simulink library "simgens"  (Simulink 6.0)
settings: Solver=ode45  StartTime=0.0  StopTime=10.0  RelTol=1e-3
model workspace (MAT data in the model file):
  libCache.blocksTree = {{'simgens', {'Band-Limited White Noise'; 'Chirp Signal'; 'Clock'; 'Constant'; 'Counter Free-Running'; 'Counter Limited'; 'Digital Clock'; 'From File'; 'From Workspace'; 'Ground'; 'Pulse Generator'; 'Ramp'; 'Random Number'; 'Repeating Sequence'; 'Repeating Sequence Interpolated'; 'Repeating Sequence Stair'; 'Signal Builder'; 'Signal Generator'; 'Sine Wave'; 'Step'; 'Uniform Random Number'}}}
  libCache.blockNames{1} = 'simgens'
  libCache.blockNames{2} = 'simgens/Band-Limited
    | White Noise'
  libCache.blockNames{3} = 'simgens/Chirp Signal'
  libCache.blockNames{4} = 'simgens/Clock'
  libCache.blockNames{5} = 'simgens/Constant'
  libCache.blockNames{6} = 'simgens/Counter
    | Free-Running'
  libCache.blockNames{7} = 'simgens/Counter
    | Limited'
  libCache.blockNames{8} = 'simgens/Digital Clock'
  libCache.blockNames{9} = 'simgens/From File'
  libCache.blockNames{10} = 'simgens/From
    | Workspace'
  libCache.blockNames{11} = 'simgens/Ground'
  libCache.blockNames{12} = 'simgens/Pulse
    | Generator'
  libCache.blockNames{13} = 'simgens/Ramp'
  libCache.blockNames{14} = 'simgens/Random
    | Number'
  libCache.blockNames{15} = 'simgens/Repeating
    | Sequence'
  libCache.blockNames{16} = 'simgens/Repeating
    | Sequence
    | Interpolated'
  libCache.blockNames{17} = 'simgens/Repeating
    | Sequence
    | Stair'
  libCache.blockNames{18} = 'simgens/Signal Builder'
  libCache.blockNames{19} = 'simgens/Signal
    | Generator'
  libCache.blockNames{20} = 'simgens/Sine Wave'
  libCache.blockNames{21} = 'simgens/Step'
  libCache.blockNames{22} = 'simgens/Uniform Random
    | Number'
undefined symbols (not defined in the file or in its folder): sigbuilder_block
libraries: simulink x8
PreSaveFcn:
  | iomanager('UpdateCache',bdroot(gcs))
settings Model: LibraryType=IOLibrary  Creator=weis  LastModifiedBy=andyb  ExtModeAutoUpdateStatusClock=off
settings DataIOCC: SignalLoggingName=logsOut
settings DebuggingCC: CheckExecutionContextPreStartOutputMsg=on  CheckExecutionContextRuntimeOutputMsg=on
settings SFSimCC: SFSimApplyToAllLibs=on  SFSimBuildMode=Incremental

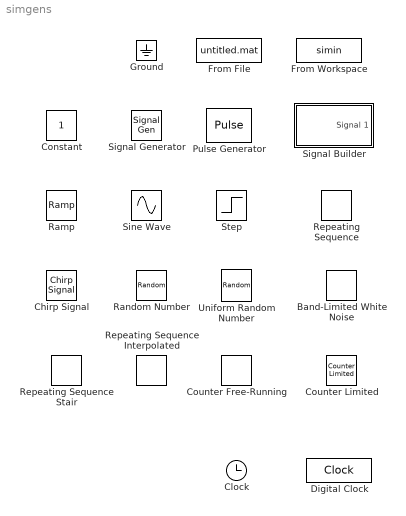
== system simgens ==
  Band-Limited White Noise : simulink/Sources/Band-Limited White Noise  IOType=siggen  Cov=[0.1]  Ts=0.1  seed=[23341]
  Chirp Signal : simulink/Sources/Chirp Signal  IOType=siggen  f1=0.1  T=100  f2=1
  Clock : Clock
      settings: IOType=siggen  Decimation=10
  Constant : Constant  IOType=siggen
  Counter Free-Running : simulink/Sources/Counter Free-Running  IOType=siggen  NumBits=16  tsamp=-1
  Counter Limited : simulink/Sources/Counter Limited  IOType=siggen  uplimit=7  tsamp=-1
  Digital Clock : DigitalClock  IOType=siggen
  From Workspace : FromWorkspace  IOType=siggen  VariableName=simin  SampleTime=0
  From File : FromFile  IOType=siggen  SampleTime=0
  Ground : Ground  IOType=siggen
  Pulse Generator : DiscretePulseGenerator  IOType=siggen  PulseType=Time based  PulseWidth=50
  Ramp : simulink/Sources/Ramp  IOType=siggen  slope=1  start=0  X0=0
  Random Number : RandomNumber  IOType=siggen  SampleTime=0
  Repeating Sequence : simulink/Sources/Repeating Sequence  IOType=siggen  rep_seq_t=[0 2]  rep_seq_y=[0 2]
  Repeating Sequence Interpolated : simulink/Sources/Repeating Sequence Interpolated  IOType=siggen  OutValues=[3 1 4 2 1].'  TimeValues=[0 0.1 0.5 0.6 1].'  LookUpMeth=Interpolation-Use End Values  tsamp=0.01  OutputDataTypeScalingMode=Specify via dialog  OutDataType=float('double')  OutScaling=2^-10
  Repeating Sequence Stair : simulink/Sources/Repeating Sequence Stair  IOType=siggen  OutValues=[3 1 4 2 1].'  tsamp=-1  OutputDataTypeScalingMode=Specify via dialog  OutDataType=float('double')  ConRadixGroup=Best Precision: Vector-wise  OutScaling=2^-12
  Signal Generator : SignalGenerator  IOType=siggen
  Signal Builder : Subsystem  Tag=STV Subsys  IOType=siggen  StartFcn=sigbuilder_block('start');  StopFcn=sigbuilder_block('stop');  ClipboardFcn=sigbuilder_block('clipboard');  PropExecContextAcrossSSBoundary=on  mask(Sigbuilder block){}
      mask help: Sigbuilder GUI
      mask init:
      | if ~strcmp(get_param(bdroot(gcbh),'SimulationStatus'),'stopped') tuvar = sigbuilder_block('maskInit'); end
      settings: CopyFcn=sigbuilder_block('copy');  DeleteFcn=sigbuilder_block('delete');  ModelCloseFcn=sigbuilder_block('modelClose');  PreSaveFcn=sigbuilder_block('preSave');  NameChangeFcn=sigbuilder_block('namechange');  OpenFcn=sigbuilder_block('open',[50 50 520 400 ]);  CloseFcn=sigbuilder_block('close');
      mask Display: plot(0,0,100,100,[10,10,40,40,10],[80,20,20,80,80],[40,10],[50,50], [40,27,10],[65,72,56],[40,25,25,10],[28,28,43,43]);
  Sine Wave : Sin  IOType=siggen  SampleTime=0
  Step : Step  IOType=siggen  SampleTime=0
  Uniform Random Number : UniformRandomNumber  IOType=siggen  SampleTime=0

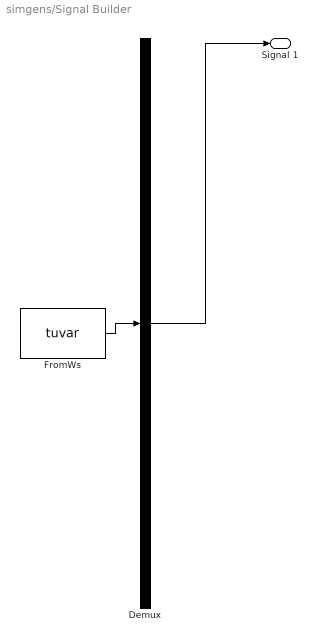
== system simgens/Signal Builder ==
  Demux : Demux  Tag=STV Demux  Outputs=1
  FromWs : FromWorkspace  Tag=STV FromWs  VariableName=tuvar  SampleTime=0  SigBuilderData=DataTag1
      SigBuilderData=|
      | channels.label = 'Signal 1'
      | channels.allXData = {[0 4 4 6 6 10]}
      | channels.allYData = {[0 0 1 1 0 0]}
      | dataSet.timeRange = [0 10]
      | dataSet.name = 'Group 1'
  Signal 1 : Outport  Tag=STV Outport
  wires:
  Demux/1 -> Signal 1/1
  FromWs/1 -> Demux/1
